simulink model "podd"  (R2020a)
settings: Solver=ode45  StartTime=0.0  StopTime=600  RelTol=1e-3  EnableMultiTasking=on
values from neighbouring files (symbols this model uses):
  A1 = str2double(get(handles.edit5,'string'))    [Gui.m]
  A2 = str2double(get(handles.edit6,'string'))    [Gui.m]
  mi1 = str2double(get(handles.edit3,'string'))    [Gui.m]
  mi2 = str2double(get(handles.edit4,'string'))    [Gui.m]
  mu1 = str2double(get(handles.edit2,'string'))    [Gui.m]
settings Model: Creator=Sandra Knezevic  LastModifiedBy=Aldin
settings DataIOCC: LimitDataPoints=on  SaveFormat=Array  ReturnWorkspaceOutputs=off
settings OptimizationCC: LifeSpan=inf
settings DebuggingCC: SFUnexpectedBacktrackingDiag=warning  SFNoUnconditionalDefaultTransitionDiag=warning  SFExecutionAtInitializationDiag=none  ArithmeticOperatorsInVariantConditions=warning
settings HardwareCC: ProdBitPerPointer=32  ProdBitPerSizeT=32  ProdBitPerPtrDiffT=32  ProdLargestAtomicFloat=None  ProdIntDivRoundTo=Undefined  ProdEndianess=Unspecified  ProdWordSize=32  ProdHWDeviceType=32-bit Generic
settings ModelReferenceCC: PropagateSignalLabelsOutOfModel=off
settings SFSimCC: SimUseLocalCustomCode=off  CustomCodeUndefinedFunction=UseInterfaceOnly
settings RTWCC: RTWUseLocalCustomCode=off
settings CodeAppCC: StateflowObjectComments=on
settings GRTTargetCC: TargetLangStandard=C89/C90 (ANSI)
settings ConfigComp: CovMetricSettings=dw  CovHtmlReporting=on  CovSaveCumulativeToWorkspaceVar=on  CovSaveSingleToWorkspaceVar=on  CovExternalEMLEnable=off

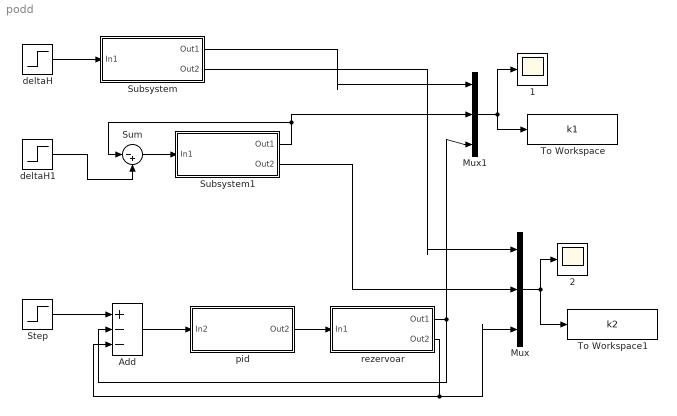
== system podd ==
  1 : Scope
  2 : Scope
  Add : Sum  Inputs=+--
  Mux : Mux  Inputs=3
  Mux1 : Mux  Inputs=3
  Step : Step  Time=0  Before=1  After=10  SampleTime=0
  Subsystem : Subsystem
  Subsystem1 : Subsystem
  Sum : Sum  Inputs=|-+
  To Workspace : ToWorkspace  VariableName=k1  SampleTime=-1
  To Workspace1 : ToWorkspace  VariableName=k2  SampleTime=-1
  deltaH : Step  After=15  SampleTime=0
  deltaH1 : Step  After=15  SampleTime=0
  pid : Subsystem
  rezervoar : Subsystem
  wires:
  deltaH/1 -> Subsystem/1(In1)
  deltaH1/1 -> Sum/2
  Sum/1 -> Subsystem1/1(In1)
  Subsystem1/1(Out1) -> Mux1/2, Sum/1
  pid/1(Out2) -> rezervoar/1(In1)
  Add/1 -> pid/1(In2)
  Step/1 -> Add/1
  rezervoar/1(Out1) -> Mux1/3, Add/2
  rezervoar/2(Out2) -> Add/3, Mux/3
  Mux1/1 -> 1/1, To Workspace/1
  Subsystem/1(Out1) -> Mux1/1
  Subsystem/2(Out2) -> Mux/1
  Subsystem1/2(Out2) -> Mux/2
  Mux/1 -> To Workspace1/1, 2/1

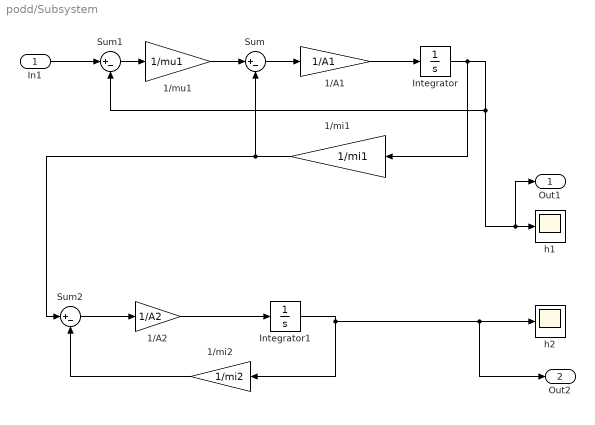
== system podd/Subsystem ==
  In1 : Inport
  1/A1 : Gain  Gain=1/A1
  1/A2 : Gain  Gain=1/A2
  1/mi1 : Gain  Gain=1/mi1
  1/mi2 : Gain  Gain=1/mi2
  1/mu1 : Gain  Gain=1/mu1
  Integrator : Integrator  InitialCondition=1
  Integrator1 : Integrator  InitialCondition=1
  Sum : Sum  Inputs=|+-
  Sum1 : Sum  Inputs=|+-
  Sum2 : Sum  Inputs=|+-
  h1 : Scope
  h2 : Scope
  Out1 : Outport
  Out2 : Outport  Port=2
  wires:
  Integrator1/1 -> Out2/1, h2/1, 1/mi2/1
  Sum/1 -> 1/A1/1
  1/mi2/1 -> Sum2/2
  Sum1/1 -> 1/mu1/1
  1/A2/1 -> Integrator1/1
  1/mu1/1 -> Sum/1
  1/mi1/1 -> Sum/2, Sum2/1
  In1/1 -> Sum1/1
  Integrator/1 -> 1/mi1/1, Out1/1, h1/1, Sum1/2
  1/A1/1 -> Integrator/1
  Sum2/1 -> 1/A2/1

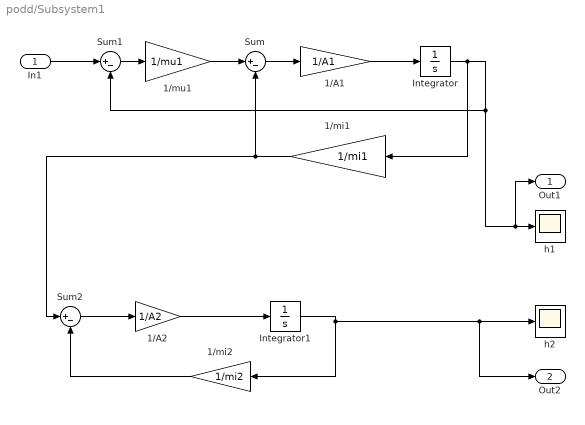
== system podd/Subsystem1 ==
  In1 : Inport
  1/A1 : Gain  Gain=1/A1
  1/A2 : Gain  Gain=1/A2
  1/mi1 : Gain  Gain=1/mi1
  1/mi2 : Gain  Gain=1/mi2
  1/mu1 : Gain  Gain=1/mu1
  Integrator : Integrator  InitialCondition=1
  Integrator1 : Integrator  InitialCondition=1
  Sum : Sum  Inputs=|+-
  Sum1 : Sum  Inputs=|+-
  Sum2 : Sum  Inputs=|+-
  h1 : Scope
  h2 : Scope
  Out1 : Outport
  Out2 : Outport  Port=2
  wires:
  Sum2/1 -> 1/A2/1
  1/A1/1 -> Integrator/1
  1/mi1/1 -> Sum/2, Sum2/1
  1/mu1/1 -> Sum/1
  Sum1/1 -> 1/mu1/1
  1/A2/1 -> Integrator1/1
  1/mi2/1 -> Sum2/2
  Integrator/1 -> 1/mi1/1, Out1/1, h1/1, Sum1/2
  In1/1 -> Sum1/1
  Integrator1/1 -> Out2/1, h2/1, 1/mi2/1
  Sum/1 -> 1/A1/1

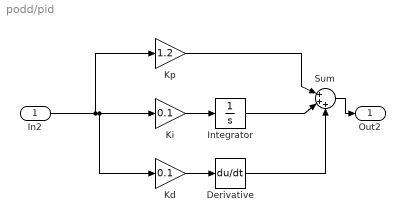
== system podd/pid ==
  In2 : Inport
  Derivative : Derivative
  Integrator : Integrator
  Kd : Gain  Gain=0.1
  Ki : Gain  Gain=0.1
  Kp : Gain  Gain=1.2
  Sum : Sum  Inputs=|+++
  Out2 : Outport
  wires:
  Kp/1 -> Sum/1
  Integrator/1 -> Sum/2
  Derivative/1 -> Sum/3
  Sum/1 -> Out2/1
  In2/1 -> Kp/1, Kd/1, Ki/1
  Ki/1 -> Integrator/1
  Kd/1 -> Derivative/1

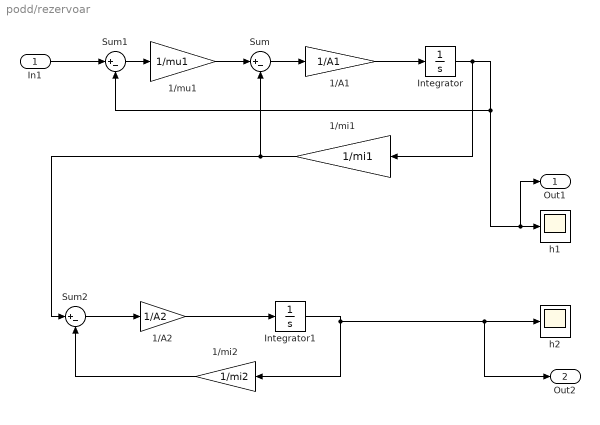
== system podd/rezervoar ==
  In1 : Inport
  1/A1 : Gain  Gain=1/A1
  1/A2 : Gain  Gain=1/A2
  1/mi1 : Gain  Gain=1/mi1
  1/mi2 : Gain  Gain=1/mi2
  1/mu1 : Gain  Gain=1/mu1
  Integrator : Integrator  InitialCondition=1
  Integrator1 : Integrator  InitialCondition=1
  Sum : Sum  Inputs=|+-
  Sum1 : Sum  Inputs=|+-
  Sum2 : Sum  Inputs=|+-
  h1 : Scope
  h2 : Scope
  Out1 : Outport
  Out2 : Outport  Port=2
  wires:
  Sum2/1 -> 1/A2/1
  1/A1/1 -> Integrator/1
  1/mi1/1 -> Sum/2, Sum2/1
  1/mu1/1 -> Sum/1
  Sum1/1 -> 1/mu1/1
  1/A2/1 -> Integrator1/1
  1/mi2/1 -> Sum2/2
  Integrator/1 -> 1/mi1/1, Out1/1, h1/1, Sum1/2
  In1/1 -> Sum1/1
  Integrator1/1 -> Out2/1, h2/1, 1/mi2/1
  Sum/1 -> 1/A1/1
